simulink model "ex3_sim1"  (R2018b)
settings: Solver=ode45  StartTime=0.0  StopTime=1.5  MaxStep=0.001  RelTol=1e-3
undefined symbols (not defined in the file): DiscIntNeverNeededParam, kawu, kd, ki, km, kp, Td, Tm, Ts
settings Model: Creator=riccardo  LastModifiedBy=riccardo

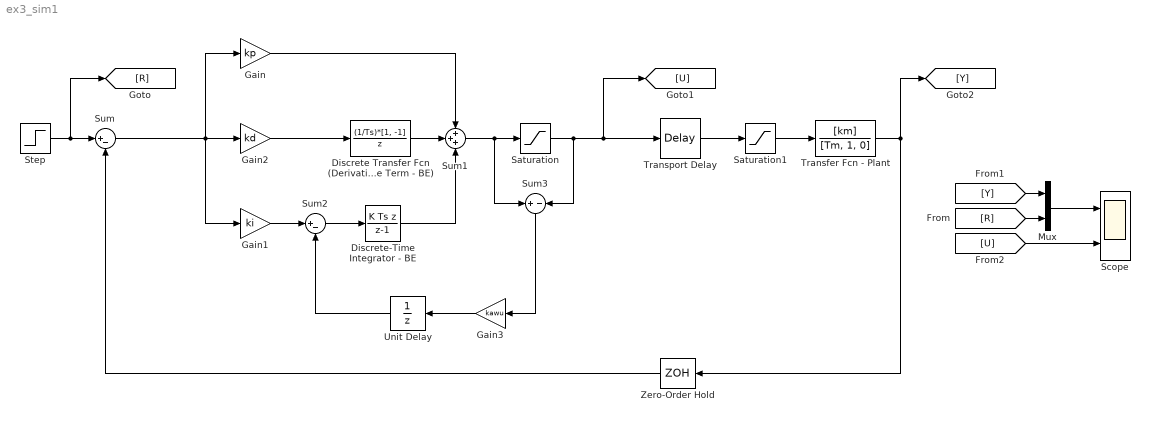
== system ex3_sim1 ==
  Discrete Transfer Fcn (Derivative Term - BE) : DiscreteTransferFcn  Numerator=(1/Ts)*[1, -1]  Denominator=[1, 0]  SampleTime=Ts
  Discrete-Time Integrator - BE : DiscreteIntegrator  IntegratorMethod=Integration: Backward Euler  SampleTime=Ts  ICPrevOutput=DiscIntNeverNeededParam  ICPrevScaledInput=DiscIntNeverNeededParam
  Gain : Gain  Gain=kp
  Gain1 : Gain  Gain=ki
  Gain2 : Gain  Gain=kd
  Gain3 : Gain  Gain=kawu
  Mux : Mux  Inputs=2
  Saturation : Saturate  UpperLimit=6  LowerLimit=-6
  Saturation1 : Saturate  UpperLimit=6  LowerLimit=-6
  Scope : Scope  NumInputPorts=2
  Step : Step  Time=0.1  SampleTime=Ts
  Sum : Sum  Inputs=|+-
  Sum1 : Sum  Inputs=+++
  Sum2 : Sum  Inputs=|+-
  Sum3 : Sum  Inputs=+-
  Transfer Fcn - Plant : TransferFcn  Numerator=[km]  Denominator=[Tm, 1, 0]
  Transport Delay : TransportDelay  DelayTime=Td
  Unit Delay : UnitDelay  SampleTime=Ts
  Zero-Order Hold : ZeroOrderHold  SampleTime=Ts
  wires:
  Transport Delay/1 -> Saturation1/1
  Sum1/1 -> Sum3/1, Saturation/1
  Transfer Fcn - Plant/1 -> [Y], Zero-Order Hold/1
  Zero-Order Hold/1 -> Sum/2
  Sum/1 -> Gain/1, Gain1/1, Gain2/1
  Step/1 -> [R], Sum/1
  Mux/1 -> Scope/1
  [R] -> Mux/2
  [Y] -> Mux/1
  [U] -> Scope/2
  Gain2/1 -> Discrete Transfer Fcn (Derivative Term - BE)/1
  Discrete Transfer Fcn (Derivative Term - BE)/1 -> Sum1/2
  Discrete-Time Integrator - BE/1 -> Sum1/3
  Gain/1 -> Sum1/1
  Saturation/1 -> Sum3/2, [U], Transport Delay/1
  Gain1/1 -> Sum2/1
  Sum2/1 -> Discrete-Time Integrator - BE/1
  Sum3/1 -> Gain3/1
  Gain3/1 -> Unit Delay/1
  Saturation1/1 -> Transfer Fcn - Plant/1
  Unit Delay/1 -> Sum2/2
